simulink model "mag_schwebe_pid"  (Simulink 4.00)
settings: Solver=ode45  StartTime=0.0  StopTime=20.0  MaxStep=0.01  RelTol=1e-3
libraries: simulink3 x2
settings Model: LastModifiedBy=Brunner  BlockReductionOpt=off

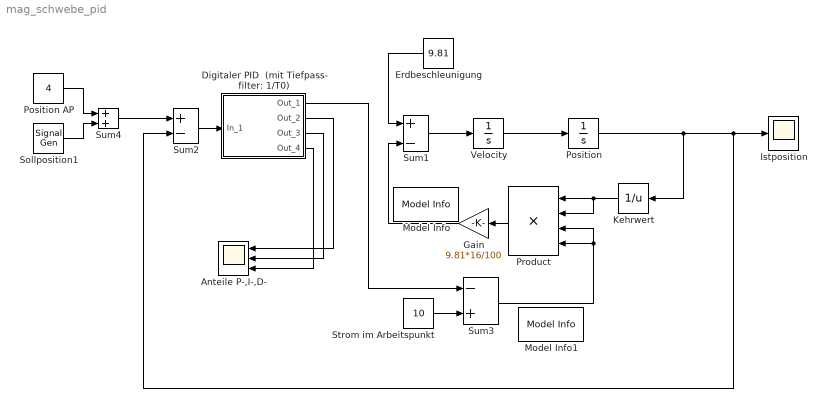
== system mag_schwebe_pid ==
  Anteile P-,I-,D- : Scope  NumInputPorts=3
      settings: TimeRange=20  YMin=-0.4~-0.1~-4  YMax=0.6~0.1~4  SaveToWorkspace=off  SaveName=ScopeData2  LimitDataPoints=on  MaxDataPoints=5000
  Digitaler PID  (mit Tiefpass- filter: 1/T0) : Subsystem  mask(PID Controller){T0=0.1, P=20, I=10, D=8}
      mask prompts: T0 "Zeitkonstante:"; P "Proportional:"; I "Integral"; D "Derivative:"
      mask help:
      | Enter expressions for proportional, integral, and derivative terms.
      | P+I/s+Ds
      settings: RTWFcnNameOpts=Auto  RTWFileNameOpts=Auto
      mask Help: This block implements a PID controller where parameters are entered for the Proportional, Integral and Derivative terms. Unmask this block to see how it works. The derivative term is implemented using a true derivative block.
      mask Display: disp('PID')
  Erdbeschleunigung : Constant  Orientation=left  Value=9.81
  Gain : Gain  Orientation=left  Gain=9.81*16/100  Multiplication=Element-wise(K.*u)  SaturateOnIntegerOverflow=on
  Istposition : Scope
      settings: TimeRange=20  YMin=3.94  YMax=4.06  SaveToWorkspace=off  SaveName=ScopeData  LimitDataPoints=on  MaxDataPoints=5000
  Kehrwert : Math  Orientation=left  Operator=reciprocal  OutputSignalType=auto
  Model Info : simulink3/Signals & Systems/Model Info  InitialBlockCM=none  BlockCM=none  Frame=off  DisplayStringWithTags=|  HorizontalTextAlignment=Center  LeftAlignmentValue=0.5  SourceBlockDiagram=mag_schwebe_pid  TagMaxNumber=20
      | Magnet-
      | kraft (norm.)
  Model Info1 : simulink3/Signals & Systems/Model Info  InitialBlockCM=none  BlockCM=none  Frame=off  DisplayStringWithTags=geregelter Spulenstrom  HorizontalTextAlignment=Center  LeftAlignmentValue=0.5  SourceBlockDiagram=mag_schwebe_pid  TagMaxNumber=20
  Position : Integrator  ExternalReset=none  InitialConditionSource=internal  InitialCondition=4  LimitOutput=off  UpperSaturationLimit=inf  LowerSaturationLimit=-inf  ShowSaturationPort=off  ShowStatePort=off  AbsoluteTolerance=auto
  Position AP : Constant  Value=4
  Product : Product  Orientation=left  Inputs=4  Multiplication=Element-wise(.*)  SaturateOnIntegerOverflow=on
  Sollposition1 : SignalGenerator  WaveForm=square  Amplitude=0.05  Frequency=0.1  Units=Hertz
  Strom im Arbeitspunkt : Constant  Value=10
  Sum1 : Sum  Inputs=+-  SaturateOnIntegerOverflow=on
  Sum2 : Sum  Inputs=+-  SaturateOnIntegerOverflow=on
  Sum3 : Sum  Inputs=-+  SaturateOnIntegerOverflow=on
  Sum4 : Sum  Inputs=++  SaturateOnIntegerOverflow=on
  Velocity : Integrator  ExternalReset=none  InitialConditionSource=internal  InitialCondition=0  LimitOutput=off  UpperSaturationLimit=inf  LowerSaturationLimit=-inf  ShowSaturationPort=off  ShowStatePort=off  AbsoluteTolerance=auto
  wires:
  Gain/1 -> Sum1/2
  Sum1/1 -> Velocity/1
  Velocity/1 -> Position/1
  Position/1 -> Kehrwert/1, Istposition/1, Sum2/2
  Product/1 -> Gain/1
  Kehrwert/1 -> Product/1, Product/2
  Position AP/1 -> Sum4/1
  Sollposition1/1 -> Sum4/2
  Erdbeschleunigung/1 -> Sum1/1
  Sum4/1 -> Sum2/1
  Sum2/1 -> Digitaler PID  (mit Tiefpass- filter: 1/T0)/1(In_1)
  Digitaler PID  (mit Tiefpass- filter: 1/T0)/2(Out_2) -> Anteile P-,I-,D-/1
  Digitaler PID  (mit Tiefpass- filter: 1/T0)/3(Out_3) -> Anteile P-,I-,D-/2
  Digitaler PID  (mit Tiefpass- filter: 1/T0)/4(Out_4) -> Anteile P-,I-,D-/3
  Strom im Arbeitspunkt/1 -> Sum3/2
  Digitaler PID  (mit Tiefpass- filter: 1/T0)/1(Out_1) -> Sum3/1
  Sum3/1 -> Product/3, Product/4

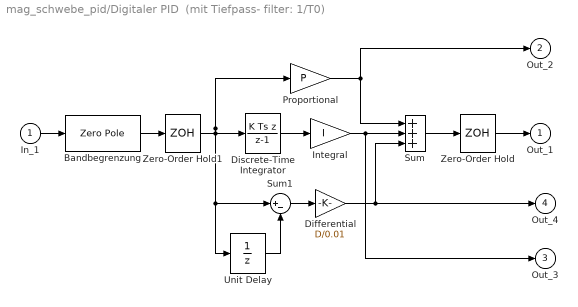
== system mag_schwebe_pid/Digitaler PID  (mit Tiefpass- filter: 1/T0) ==
  In_1 : Inport  Port=1
  Bandbegrenzung : ZeroPole  Zeros=[]  Poles=[-1/T0]  Gain=[1/T0]  AbsoluteTolerance=auto
  Differential : Gain  Gain=D/0.01  Multiplication=Element-wise(K.*u)  SaturateOnIntegerOverflow=on
  Discrete-Time Integrator : DiscreteIntegrator  IntegratorMethod=BackwardEuler  ExternalReset=none  InitialConditionSource=internal  InitialCondition=0  LimitOutput=off  UpperSaturationLimit=inf  LowerSaturationLimit=-inf  ShowSaturationPort=off  ShowStatePort=off  SampleTime=0.01
  Integral : Gain  Gain=I  Multiplication=Element-wise(K.*u)  SaturateOnIntegerOverflow=on
  Proportional : Gain  Gain=P  Multiplication=Element-wise(K.*u)  SaturateOnIntegerOverflow=on
  Sum : Sum  Inputs=+++  SaturateOnIntegerOverflow=on
  Sum1 : Sum  Inputs=|+-  SaturateOnIntegerOverflow=on
  Unit Delay : UnitDelay  X0=0  SampleTime=0.01
  Zero-Order Hold : ZeroOrderHold  SampleTime=0.01
  Zero-Order Hold1 : ZeroOrderHold  SampleTime=0.01
  Out_1 : Outport  Port=1  InitialOutput=0
  Out_2 : Outport  Port=2  InitialOutput=0
  Out_3 : Outport  Port=3  InitialOutput=0
  Out_4 : Outport  Port=4  InitialOutput=0
  wires:
  Differential/1 -> Sum/3, Out_4/1
  In_1/1 -> Bandbegrenzung/1
  Bandbegrenzung/1 -> Zero-Order Hold1/1
  Sum/1 -> Zero-Order Hold/1
  Zero-Order Hold/1 -> Out_1/1
  Zero-Order Hold1/1 -> Discrete-Time Integrator/1, Sum1/1, Unit Delay/1, Proportional/1
  Proportional/1 -> Sum/1, Out_2/1
  Sum1/1 -> Differential/1
  Unit Delay/1 -> Sum1/2
  Discrete-Time Integrator/1 -> Integral/1
  Integral/1 -> Sum/2, Out_3/1
